simulink model "HAPSRAV_ENERGY_SIM"  (R2017a)
settings: Solver=ode1  StartTime=0.0  StopTime=tfin  FixedStep=dT  MaxStep=dT*10  MinStep=dT  RelTol=1e-3
libraries: hapsrav_library x2
settings Model: SimulationMode=accelerator  Creator=jack.marriott  LastModifiedBy=marriott
settings SolverCC: InitialStep=dT  ZeroCrossControl=EnableAll
settings DataIOCC: SaveOutput=off  SignalLogging=off  DSMLogging=off  ReturnWorkspaceOutputs=on  ReturnWorkspaceOutputsName=ksim
settings OptimizationCC: DefaultParameterBehavior=Inlined  PassReuseOutputArgsThreshold=0
settings DebuggingCC: RTPrefix=none  ReadBeforeWriteMsg=DisableAll  WriteAfterWriteMsg=DisableAll  WriteAfterReadMsg=DisableAll  MultiTaskDSMMsg=none  ParameterTunabilityLossMsg=error
settings HardwareCC: TargetBitPerPointer=64  TargetBitPerSizeT=64  TargetBitPerPtrDiffT=64  TargetLongLongMode=on  TargetIntDivRoundTo=Zero  TargetEndianess=LittleEndian  TargetWordSize=64  TargetHWDeviceType=MATLAB Host  ProdEqTarget=off
settings ModelReferenceCC: UpdateModelReferenceTargets=IfOutOfDate  ModelReferenceMinAlgLoopOccurrences=on
settings SFSimCC: SimUserSources=date_vec.c  SFSimEcho=off  MATLABDynamicMemAlloc=off
settings RTWCC: SystemTargetFile=rsim.tlc  TemplateMakefile=rsim_default_tmf  Description=Rapid Simulation Target  GenerateReport=on  RTWUseSimCustomCode=on  CustomSource=date_vec.c  LaunchReport=on
settings CodeAppCC: ForceParamTrailComments=on  OperatorAnnotations=on  MATLABSourceComments=on
settings TargetCC: TargetLangStandard=C99 (ISO)  ParMdlRefBuildCompliant=on  ConcurrentExecutionCompliant=on  GeneratePreprocessorConditionals=Use local settings  MatFileLogging=on

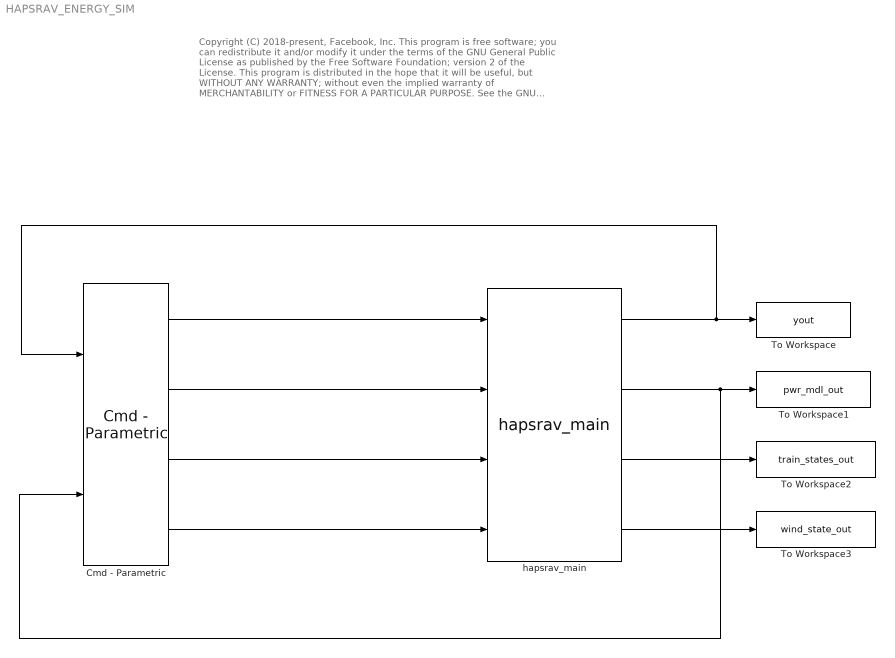
== system HAPSRAV_ENERGY_SIM ==
  note: Copyright (C) 2018-present, Facebook, Inc.
      |
      | This program is free software; you can redistribute it and/or modify
      | it under the terms of the GNU General Public License as published by
      | the Free Software Foundation; version 2 of the License.
      |
      | This program is distributed in the hope that it will be useful,
      | but WITHOUT ANY WARRANTY; without even the implied warranty of
      | MERCHANTABILITY or FITNESS FOR A PARTICULAR PURPOSE. See the
      | GNU General Public License for more details.
      |
      | You should have received a copy of the GNU General Public License along
      | with this program; if not, write to the Free Software Foundation, Inc.,
      | 51 Franklin Street, Fifth Floor, Boston, MA 02110-1301 USA.
  Cmd - Parametric : hapsrav_library/Cmd - Parametric
  To Workspace : ToWorkspace  VariableName=yout  SaveFormat=Structure  SampleTime=-1
  To Workspace1 : ToWorkspace  VariableName=pwr_mdl_out  SaveFormat=Structure  SampleTime=-1
  To Workspace2 : ToWorkspace  VariableName=train_states_out  SaveFormat=Structure  SampleTime=-1
  To Workspace3 : ToWorkspace  VariableName=wind_state_out  SaveFormat=Structure  SampleTime=-1
  hapsrav_main : hapsrav_library/hapsrav_main
  wires:
  hapsrav_main/1 -> Cmd - Parametric/1, To Workspace/1
  hapsrav_main/2 -> Cmd - Parametric/2, To Workspace1/1
  Cmd - Parametric/1 -> hapsrav_main/1
  Cmd - Parametric/2 -> hapsrav_main/2
  Cmd - Parametric/3 -> hapsrav_main/3
  Cmd - Parametric/4 -> hapsrav_main/4
  hapsrav_main/3 -> To Workspace2/1
  hapsrav_main/4 -> To Workspace3/1
